simulink model "COVID_mod"  (R2019b)
settings: Solver=ode4  StartTime=0.0  StopTime=365  FixedStep=1  MaxStep=1e-2  RelTol=1e-3
values from neighbouring files (symbols this model uses):
  D_init = 0    [covid.m]
  E_init = 20 * I_init    [covid.m]
  I_init = n    [covid.m]
  matA = [0 0 0 0 0 ... (first row only)    [covid.m]
  matB1 = [sigma*beta/N; -sigma*beta/N; 0; 0; 0]    [covid.m]
  matB2 = [xi; 0; 0; -xi; 0]    [covid.m]
  matB3 = [-beta/N; beta/N; 0; 0; 0]    [covid.m]
  matB3Hi = matB3*Hi    [covid.m]
  matB3Lo = matB3*Lo    [covid.m]
  matC = eye( 5 )    [covid.m]
  R_init = 0    [covid.m]
  S_init = N - I_init - E_init - D_init - R_init    [covid.m]
  tau_sigmapost = str2double( get( handles.tau_sigmapost, 'String' ) )    [covid.m]
  tau_sigmapre = str2double( get( handles.tau_sigmapre, 'String' ) )    [covid.m]
  tau_xi = str2double( get( handles.tau_xi, 'String' ) )    [covid.m]
libraries: simulink x3
settings Model: Creator=markng  LastModifiedBy=markng
settings DataIOCC: OutputSaveName=out
settings DebuggingCC: AlgebraicLoopMsg=none  ArtificialAlgebraicLoopMsg=none

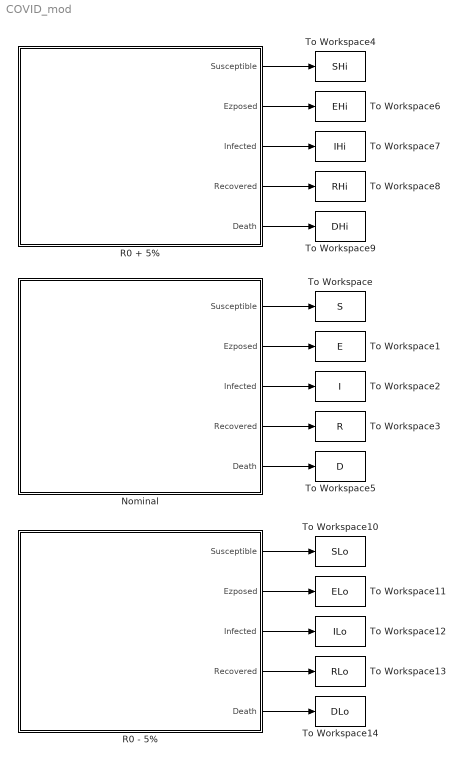
== system COVID_mod ==
  Nominal : Subsystem
  R0 + 5% : Subsystem
  R0 - 5% : Subsystem
  To Workspace : ToWorkspace  VariableName=S  SaveFormat=Timeseries  SampleTime=-1
  To Workspace1 : ToWorkspace  VariableName=E  SaveFormat=Timeseries  SampleTime=-1
  To Workspace10 : ToWorkspace  VariableName=SLo  SaveFormat=Timeseries  SampleTime=-1
  To Workspace11 : ToWorkspace  VariableName=ELo  SaveFormat=Timeseries  SampleTime=-1
  To Workspace12 : ToWorkspace  VariableName=ILo  SaveFormat=Timeseries  SampleTime=-1
  To Workspace13 : ToWorkspace  VariableName=RLo  SaveFormat=Timeseries  SampleTime=-1
  To Workspace14 : ToWorkspace  VariableName=DLo  SaveFormat=Timeseries  SampleTime=-1
  To Workspace2 : ToWorkspace  VariableName=I  SaveFormat=Timeseries  SampleTime=-1
  To Workspace3 : ToWorkspace  VariableName=R  SaveFormat=Timeseries  SampleTime=-1
  To Workspace4 : ToWorkspace  VariableName=SHi  SaveFormat=Timeseries  SampleTime=-1
  To Workspace5 : ToWorkspace  VariableName=D  SaveFormat=Timeseries  SampleTime=-1
  To Workspace6 : ToWorkspace  VariableName=EHi  SaveFormat=Timeseries  SampleTime=-1
  To Workspace7 : ToWorkspace  VariableName=IHi  SaveFormat=Timeseries  SampleTime=-1
  To Workspace8 : ToWorkspace  VariableName=RHi  SaveFormat=Timeseries  SampleTime=-1
  To Workspace9 : ToWorkspace  VariableName=DHi  SaveFormat=Timeseries  SampleTime=-1
  wires:
  Nominal/1(Susceptible) -> To Workspace/1
  Nominal/2(Ezposed) -> To Workspace1/1
  Nominal/3(Infected) -> To Workspace2/1
  Nominal/4(Recovered) -> To Workspace3/1
  Nominal/5(Death) -> To Workspace5/1
  R0 + 5%/1(Susceptible) -> To Workspace4/1
  R0 + 5%/2(Ezposed) -> To Workspace6/1
  R0 + 5%/3(Infected) -> To Workspace7/1
  R0 + 5%/4(Recovered) -> To Workspace8/1
  R0 + 5%/5(Death) -> To Workspace9/1
  R0 - 5%/1(Susceptible) -> To Workspace10/1
  R0 - 5%/2(Ezposed) -> To Workspace11/1
  R0 - 5%/3(Infected) -> To Workspace12/1
  R0 - 5%/4(Recovered) -> To Workspace13/1
  R0 - 5%/5(Death) -> To Workspace14/1

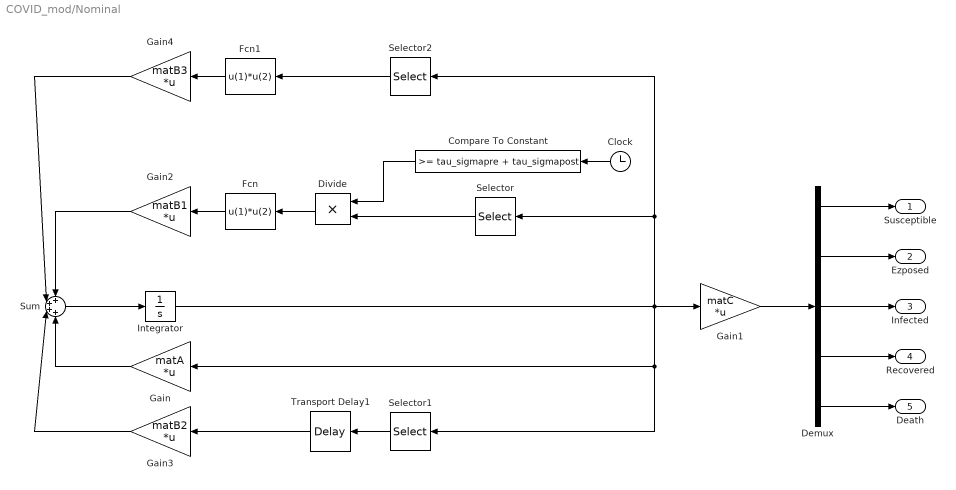
== system COVID_mod/Nominal ==
  Clock : Clock
  Compare To Constant : simulink/Logic and Bit Operations/Compare To Constant  relop=>=  const=tau_sigmapre + tau_sigmapost  OutDataTypeStr=boolean
  Demux : Demux  Outputs=5
  Divide : Product  Inputs=**
  Fcn : Fcn  Expr=u(1)*u(2)
  Fcn1 : Fcn  Expr=u(1)*u(2)
  Gain : Gain  Gain=matA  Multiplication=Matrix(K*u)
  Gain1 : Gain  Gain=matC  Multiplication=Matrix(K*u)
  Gain2 : Gain  Gain=matB1  Multiplication=Matrix(K*u)
  Gain3 : Gain  Gain=matB2  Multiplication=Matrix(K*u)
  Gain4 : Gain  Gain=matB3  Multiplication=Matrix(K*u)
  Integrator : Integrator  InitialCondition=[S_init E_init I_init R_init D_init]'  LimitOutput=on  LowerSaturationLimit=[0 0 0 0 0]'
  Selector : Selector  InputPortWidth=5  IndexOptions=Index vector (dialog)  Indices=[1 3]  OutputSizes=1
  Selector1 : Selector  InputPortWidth=5  IndexOptions=Index vector (dialog)  Indices=[4]  OutputSizes=1
  Selector2 : Selector  InputPortWidth=5  IndexOptions=Index vector (dialog)  Indices=[1 3]  OutputSizes=1
  Sum : Sum  Inputs=++++
  Transport Delay1 : TransportDelay  DelayTime=tau_xi
  Susceptible : Outport
  Ezposed : Outport  Port=2
  Infected : Outport  Port=3
  Recovered : Outport  Port=4
  Death : Outport  Port=5
  wires:
  Gain2/1 -> Sum/1
  Sum/1 -> Integrator/1
  Gain3/1 -> Sum/3
  Divide/1 -> Fcn/1
  Transport Delay1/1 -> Gain3/1
  Fcn1/1 -> Gain4/1
  Gain4/1 -> Sum/2
  Selector2/1 -> Fcn1/1
  Compare To Constant/1 -> Divide/1
  Selector/1 -> Divide/2
  Selector1/1 -> Transport Delay1/1
  Fcn/1 -> Gain2/1
  Clock/1 -> Compare To Constant/1
  Gain/1 -> Sum/4
  Integrator/1 -> Gain/1, Selector1/1, Gain1/1, Selector/1, Selector2/1
  Demux/2 -> Ezposed/1
  Demux/3 -> Infected/1
  Demux/4 -> Recovered/1
  Demux/5 -> Death/1
  Demux/1 -> Susceptible/1
  Gain1/1 -> Demux/1

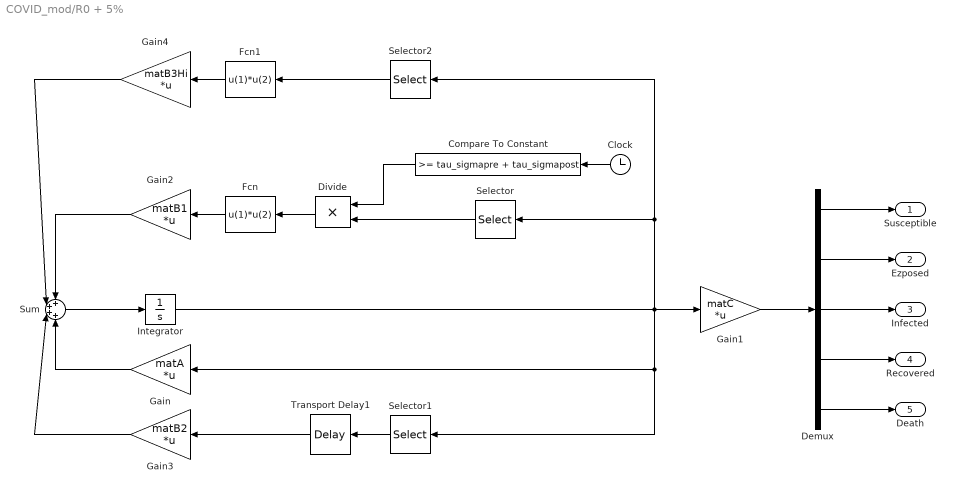
== system COVID_mod/R0 + 5% ==
  Clock : Clock
  Compare To Constant : simulink/Logic and Bit Operations/Compare To Constant  relop=>=  const=tau_sigmapre + tau_sigmapost  OutDataTypeStr=boolean
  Demux : Demux  Outputs=5
  Divide : Product  Inputs=**
  Fcn : Fcn  Expr=u(1)*u(2)
  Fcn1 : Fcn  Expr=u(1)*u(2)
  Gain : Gain  Gain=matA  Multiplication=Matrix(K*u)
  Gain1 : Gain  Gain=matC  Multiplication=Matrix(K*u)
  Gain2 : Gain  Gain=matB1  Multiplication=Matrix(K*u)
  Gain3 : Gain  Gain=matB2  Multiplication=Matrix(K*u)
  Gain4 : Gain  Gain=matB3Hi  Multiplication=Matrix(K*u)
  Integrator : Integrator  InitialCondition=[S_init E_init I_init R_init D_init]'  LimitOutput=on  LowerSaturationLimit=[0 0 0 0 0]'
  Selector : Selector  InputPortWidth=5  IndexOptions=Index vector (dialog)  Indices=[1 3]  OutputSizes=1
  Selector1 : Selector  InputPortWidth=5  IndexOptions=Index vector (dialog)  Indices=[4]  OutputSizes=1
  Selector2 : Selector  InputPortWidth=5  IndexOptions=Index vector (dialog)  Indices=[1 3]  OutputSizes=1
  Sum : Sum  Inputs=++++
  Transport Delay1 : TransportDelay  DelayTime=tau_xi
  Susceptible : Outport
  Ezposed : Outport  Port=2
  Infected : Outport  Port=3
  Recovered : Outport  Port=4
  Death : Outport  Port=5
  wires:
  Demux/2 -> Ezposed/1
  Gain3/1 -> Sum/3
  Demux/1 -> Susceptible/1
  Fcn/1 -> Gain2/1
  Gain4/1 -> Sum/2
  Clock/1 -> Compare To Constant/1
  Demux/5 -> Death/1
  Selector/1 -> Divide/2
  Transport Delay1/1 -> Gain3/1
  Gain2/1 -> Sum/1
  Compare To Constant/1 -> Divide/1
  Gain1/1 -> Demux/1
  Gain/1 -> Sum/4
  Sum/1 -> Integrator/1
  Fcn1/1 -> Gain4/1
  Divide/1 -> Fcn/1
  Demux/3 -> Infected/1
  Selector1/1 -> Transport Delay1/1
  Selector2/1 -> Fcn1/1
  Demux/4 -> Recovered/1
  Integrator/1 -> Gain/1, Selector1/1, Gain1/1, Selector/1, Selector2/1

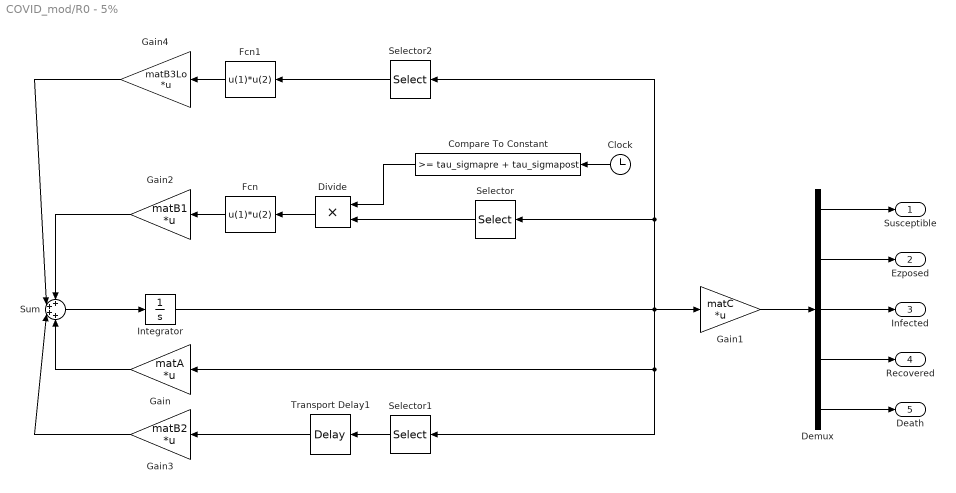
== system COVID_mod/R0 - 5% ==
  Clock : Clock
  Compare To Constant : simulink/Logic and Bit Operations/Compare To Constant  relop=>=  const=tau_sigmapre + tau_sigmapost  OutDataTypeStr=boolean
  Demux : Demux  Outputs=5
  Divide : Product  Inputs=**
  Fcn : Fcn  Expr=u(1)*u(2)
  Fcn1 : Fcn  Expr=u(1)*u(2)
  Gain : Gain  Gain=matA  Multiplication=Matrix(K*u)
  Gain1 : Gain  Gain=matC  Multiplication=Matrix(K*u)
  Gain2 : Gain  Gain=matB1  Multiplication=Matrix(K*u)
  Gain3 : Gain  Gain=matB2  Multiplication=Matrix(K*u)
  Gain4 : Gain  Gain=matB3Lo  Multiplication=Matrix(K*u)
  Integrator : Integrator  InitialCondition=[S_init E_init I_init R_init D_init]'  LimitOutput=on  LowerSaturationLimit=[0 0 0 0 0]'
  Selector : Selector  InputPortWidth=5  IndexOptions=Index vector (dialog)  Indices=[1 3]  OutputSizes=1
  Selector1 : Selector  InputPortWidth=5  IndexOptions=Index vector (dialog)  Indices=[4]  OutputSizes=1
  Selector2 : Selector  InputPortWidth=5  IndexOptions=Index vector (dialog)  Indices=[1 3]  OutputSizes=1
  Sum : Sum  Inputs=++++
  Transport Delay1 : TransportDelay  DelayTime=tau_xi
  Susceptible : Outport
  Ezposed : Outport  Port=2
  Infected : Outport  Port=3
  Recovered : Outport  Port=4
  Death : Outport  Port=5
  wires:
  Divide/1 -> Fcn/1
  Demux/1 -> Susceptible/1
  Transport Delay1/1 -> Gain3/1
  Demux/3 -> Infected/1
  Gain2/1 -> Sum/1
  Compare To Constant/1 -> Divide/1
  Fcn1/1 -> Gain4/1
  Gain4/1 -> Sum/2
  Selector2/1 -> Fcn1/1
  Demux/4 -> Recovered/1
  Gain/1 -> Sum/4
  Selector1/1 -> Transport Delay1/1
  Clock/1 -> Compare To Constant/1
  Gain1/1 -> Demux/1
  Demux/2 -> Ezposed/1
  Gain3/1 -> Sum/3
  Sum/1 -> Integrator/1
  Fcn/1 -> Gain2/1
  Demux/5 -> Death/1
  Integrator/1 -> Gain/1, Selector1/1, Gain1/1, Selector/1, Selector2/1
  Selector/1 -> Divide/2
